simulink model "PDcontrol"  (R2021a)
settings: Solver=FixedStepAuto  StartTime=0.0  StopTime=5  FixedStep=0.001  RelTol=1e-3
settings Model: Creator=negin  LastModifiedBy=negin

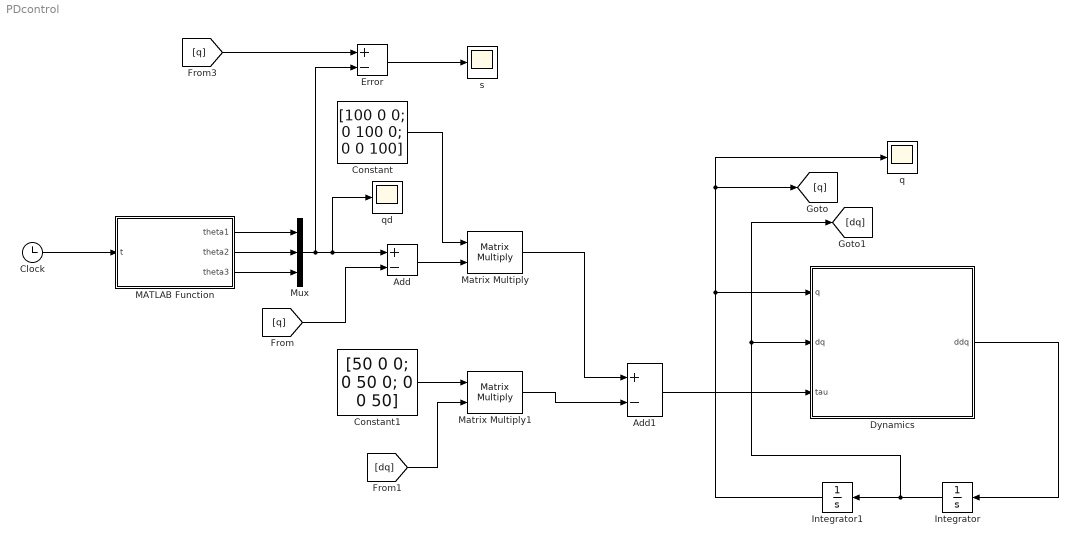
== system PDcontrol ==
  Add : Sum  Inputs=+-
  Add1 : Sum  Inputs=+-
  Clock : Clock
      settings: Decimation=5
  Constant : Constant  Value=[100 0 0; 0 100 0; 0 0 100]
  Constant1 : Constant  Value=[50 0 0; 0 50 0; 0 0 50]  VectorParams1D=off
  Dynamics : MATLAB Function  TreatAsAtomicUnit=on
  Error : Sum  Inputs=+-
  Integrator : Integrator  InitialCondition=[0; 0; 0]
  Integrator1 : Integrator  InitialCondition=[0; 0; 0]
  MATLAB Function : MATLAB Function  TreatAsAtomicUnit=on
  Matrix Multiply : Product  Multiplication=Matrix(*)
  Matrix Multiply1 : Product  Multiplication=Matrix(*)
  Mux : Mux  Inputs=3
  q : Scope
  qd : Scope
  s : Scope
  wires:
  Dynamics/1(ddq) -> Integrator/1
  Integrator/1 -> Dynamics/2(dq), [dq], Integrator1/1
  Integrator1/1 -> Dynamics/1(q), [q], q/1
  MATLAB Function/1(theta1) -> Mux/1
  Clock/1 -> MATLAB Function/1(t)
  MATLAB Function/2(theta2) -> Mux/2
  MATLAB Function/3(theta3) -> Mux/3
  Mux/1 -> Error/2, qd/1, Add/1
  [q] -> Add/2
  Add/1 -> Matrix Multiply/2
  Constant/1 -> Matrix Multiply/1
  Constant1/1 -> Matrix Multiply1/1
  [dq] -> Matrix Multiply1/2
  Matrix Multiply1/1 -> Add1/2
  Matrix Multiply/1 -> Add1/1
  Add1/1 -> Dynamics/3(tau)
  [q] -> Error/1
  Error/1 -> s/1

== matlab function PDcontrol/MATLAB Function ==
  data: theta1 output; t input; theta2 output; theta3 output
function [theta1, theta2, theta3] = desiredTraj(t)
theta1 = 0.1309*t^2 + 0.0147*t^3 - 0.0085*t^4 + 0.0007*t^5;
theta2 = 0.1309*t^2 - 0.0188*t^3 - 0.001*t^4 + 0.0002*t^5;
theta3 = 0.1309*t^2 + 0.0314*t^3 - 0.0123*t^4 + 0.001*t^5;

== matlab function PDcontrol/Dynamics ==
  data: q input; ddq output; dq input; tau input
function ddq = RobotDynamics(q, dq, tau)

m1 = 1;
m2 = 1;
m3 = 1;

l1 = 1;
l2 = 1;
l3 = 1;

r1 = l1/2;
r2 = l2/2;
r3 = l3/2;

R1 = 0.05;
R2 = 0.05;
R3 = 0.05;

g = 0;

a1 = m2*r2^2 + m3*l2^2;
a2 = m3*r3^2;
a3 = m3*r3*l2;
b1 = (m2*r2 + m3*l2)*g;
b2 = m3*r3*g;
I1 = 0.5*m1*R1^2;
I2 = 0.5*m2*R2^2;
I3 = 0.5*m3*R3^2;

M11 = a1*cos(q(2))^2 + a2*cos(q(2) + q(3))^2 + 2*a3*cos(q(2))*cos(q(2) + q(3)) + I1;
M12 = 0; 
M13 = 0; 
M21 = 0; 
M31 = 0;
M22 = a1 + a2 + 2*a3*cos(q(3)) + I2;
M23 = a2 + a3*cos(q(3));
M32 = a2 + a3*cos(q(3));
M33 = a2 + I3;
M = [M11 M12 M13; M21 M22 M23; M31 M32 M33];

C11 = -0.5*a1*dq(2)*sin(2*q(2)) - 0.5*a2*(dq(2) + dq(3))*sin(2*q(2) + 2*q(3))...
    - a3*dq(2)*sin(2*q(2) + q(3)) - a3*dq(3)*cos(q(2))*sin(q(2) + q(3));
C12 = -0.5*a1*dq(1)*sin(2*q(2)) - 0.5*a2*dq(1)*sin(2*q(2) + 2*q(3)) - ...
    a3*dq(1)*sin(2*q(2) + q(3));
C13 = -0.5*a2*dq(1)*sin(2*q(2) + 2*q(3)) - a3*dq(1)*cos(q(2))*sin(q(2) + q(3));
C21 = -C12;
C22 = -a3*dq(3)*sin(q(3));
C23 = -a3*(dq(2) + dq(3))*sin(q(3));
C31 = -C13;
C32 = a3*dq(2)*sin(q(3));
C33 = 0;
C = [C11 C12 C13; C21 C22 C23; C31 C32 C33];

G11 = 0;
G21 = m2*l2*sin(q(2))*g/2 - m3*l3*sin(q(2) + q(3))*g/2 - m3*l2*sin(q(2))*g;
G31 = -m3*l3*sin(q(2) + q(3))*g/2;
G = [G11; G21; G31];

ddq = inv(M)*(tau - C*dq - G);
end
